simulink model "ScriptSimulinkVersion"  (R2023a)
settings: Solver=VariableStepAuto  StartTime=0.0  StopTime=t(end)  RelTol=1e-3
values from neighbouring files (symbols this model uses):
  Af = 2.2    [GPT_TrailerModelv3.m]
  Bx = 8    [GPT_TrailerModelv3.m]
  Bx_cap = 6    [GPT_TrailerModelv3.m]
  Cd = 0.8    [GPT_TrailerModelv3.m]
  Crr = 0.015    [GPT_TrailerModelv3.m]
  Cseat = diag([2e3, 8e3, 1.2e4])    [GPT_TrailerModelv3.m]
  ctc = 4.0e3    (= 4000)    [GPT_TrailerModelv3.m]
  Cx = 1.5    [GPT_TrailerModelv3.m]
  Cy = 7.5e4    (= 75000)    [GPT_TrailerModelv3.m]
  CyawM = 400    [GPT_TrailerModelv3.m]
  Dx = 0.8*2500    (= 2000)    [GPT_TrailerModelv3.m]
  epsv = 0.2    [GPT_TrailerModelv3.m]
  Ex = 0.0    (= 0)    [GPT_TrailerModelv3.m]
  g = 9.81    [GPT_TrailerModelv3.m]
  IAF = diag([20, 40, 40])    [GPT_TrailerModelv3.m]
  IB = diag([450, 2200, 2500])    [GPT_TrailerModelv3.m]
  Jw = 1.8    [GPT_TrailerModelv3.m]
  Kseat = diag([2e5, 5e5, 6e4])    [GPT_TrailerModelv3.m]
  ktc = 1.2e5    (= 120000)    [GPT_TrailerModelv3.m]
  mAF = 100    [GPT_TrailerModelv3.m]
  mAR = 110    [GPT_TrailerModelv3.m]
  mB = 1200    [GPT_TrailerModelv3.m]
  mu = 1.0    (= 1)    [GPT_TrailerModelv3.m]
  r_F_L_B = [axleF_x; +trackF/2; seat_zB]    [GPT_TrailerModelv3.m]
  r_F_R_B = [axleF_x; -trackF/2; seat_zB]    [GPT_TrailerModelv3.m]
  r_LF_A = [0; +trackF/2; 0]    [GPT_TrailerModelv3.m]
  r_LR_A = [0; +trackR/2; 0]    [GPT_TrailerModelv3.m]
  r_R_L_B = [axleR_x; +trackR/2; seat_zB]    [GPT_TrailerModelv3.m]
  r_R_R_B = [axleR_x; -trackR/2; seat_zB]    [GPT_TrailerModelv3.m]
  r_RF_A = [0; -trackF/2; 0]    [GPT_TrailerModelv3.m]
  r_RR_A = [0; -trackR/2; 0]    [GPT_TrailerModelv3.m]
  rho = 1.225    [GPT_TrailerModelv3.m]
  Rw = 0.35    [GPT_TrailerModelv3.m]
  tau_sync = 0.4    [GPT_TrailerModelv3.m]
  Tloss_c = 0.01    [GPT_TrailerModelv3.m]
  v_sync_on = 0.5    [GPT_TrailerModelv3.m]
  vblend = 0.5    [GPT_TrailerModelv3.m]
  Wind_E = [0;0;0]    [GPT_TrailerModelv3.m]
  x0 = [ rB0 ... (first row only)    [GPT_TrailerModelv3.m]
undefined symbols (not defined in the file or in its folder): P
settings Model: Creator=TEOMAN  LastModifiedBy=TEOMAN

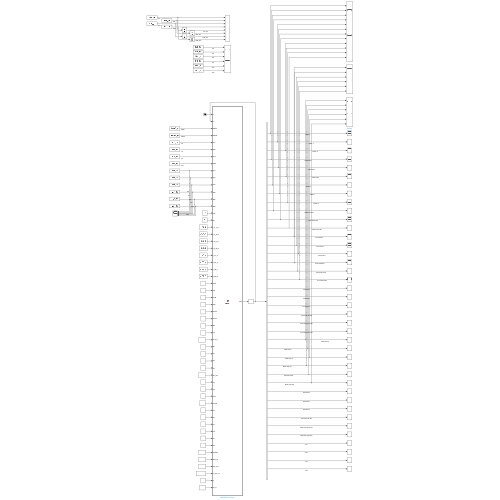
[thumbnail: Simulink's stored preview of the top-level diagram]
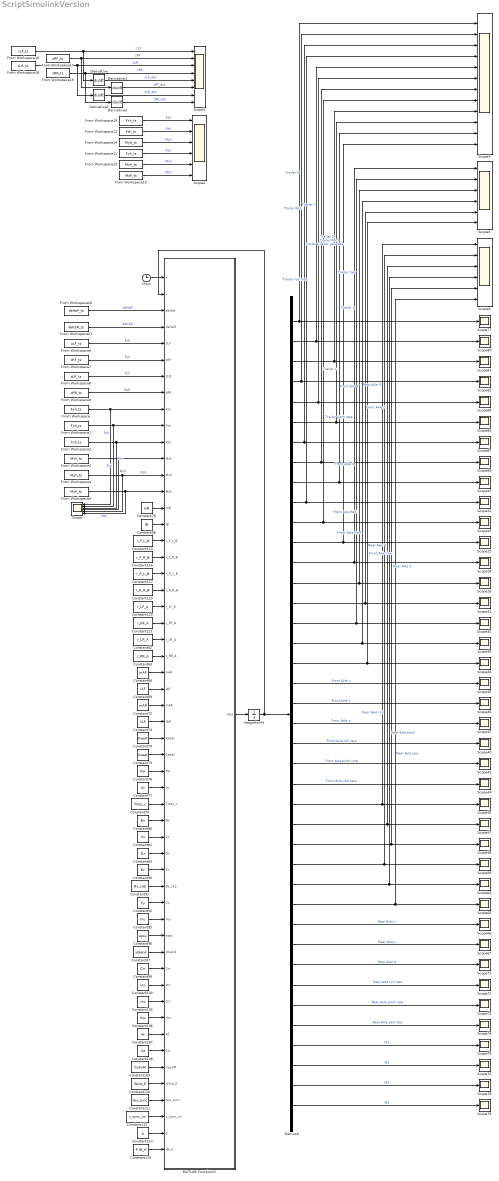
== system ScriptSimulinkVersion ==
  Clock : Clock
  Constant100 : Constant  Value=ktc
  Constant105 : Constant  Value=ctc
  Constant106 : Constant  Value=rho
  Constant107 : Constant  Value=Af
  Constant108 : Constant  Value=Cd
  Constant109 : Constant  Value=CyawM
  Constant110 : Constant  Value=Wind_E
  Constant111 : Constant  Value=tau_sync
  Constant112 : Constant  Value=v_sync_on
  Constant113 : Constant  Value=r_F_L_B
  Constant114 : Constant  Value=g
  Constant115 : Constant  Value=P.rB_H
  Constant116 : Constant  Value=r_F_R_B
  Constant117 : Constant  Value=r_R_L_B
  Constant119 : Constant  Value=r_R_R_B
  Constant120 : Constant  Value=r_LF_A
  Constant121 : Constant  Value=r_RF_A
  Constant62 : Constant  Value=r_LR_A
  Constant63 : Constant  Value=r_RR_A
  Constant66 : Constant  Value=mAF
  Constant69 : Constant  Value=IAF
  Constant72 : Constant  Value=mAR
  Constant73 : Constant  Value=IAF
  Constant74 : Constant  Value=Kseat
  Constant75 : Constant  Value=Cseat
  Constant76 : Constant  Value=Rw
  Constant77 : Constant  Value=Jw
  Constant78 : Constant  Value=mB
  Constant79 : Constant  Value=Tloss_c
  Constant80 : Constant  Value=Bx
  Constant81 : Constant  Value=Cx
  Constant83 : Constant  Value=Dx
  Constant90 : Constant  Value=Ex
  Constant91 : Constant  Value=Bx_cap
  Constant92 : Constant  Value=Cy
  Constant95 : Constant  Value=mu
  Constant96 : Constant  Value=epsv
  Constant97 : Constant  Value=vblend
  Constant98 : Constant  Value=IB
  Constant99 : Constant  Value=Crr
  Demux8 : Demux  Outputs=40
  Derivative{,1..3} (4 alike) : Derivative
  From Workspace : FromWorkspace  VariableName=Fxh_ts
  From Workspace1 : FromWorkspace  VariableName=Fyh_ts
  From Workspace10 : FromWorkspace  VariableName=Fxh_ts
  From Workspace11 : FromWorkspace  VariableName=Fyh_ts
  From Workspace12 : FromWorkspace  VariableName=Fzh_ts
  From Workspace13 : FromWorkspace  VariableName=Mxh_ts
  From Workspace14 : FromWorkspace  VariableName=Myh_ts
  From Workspace15 : FromWorkspace  VariableName=Mzh_ts
  From Workspace16 : FromWorkspace  VariableName=zLF_ts
  From Workspace17 : FromWorkspace  VariableName=zRF_ts
  From Workspace18 : FromWorkspace  VariableName=zLR_ts
  From Workspace19 : FromWorkspace  VariableName=zRR_ts
  From Workspace2 : FromWorkspace  VariableName=Fzh_ts
  From Workspace20 : FromWorkspace  VariableName=deltaF_ts
  From Workspace21 : FromWorkspace  VariableName=deltaR_ts
  From Workspace3 : FromWorkspace  VariableName=Mxh_ts
  From Workspace4 : FromWorkspace  VariableName=Myh_ts
  From Workspace5 : FromWorkspace  VariableName=Mzh_ts
  From Workspace6 : FromWorkspace  VariableName=zLF_ts
  From Workspace7 : FromWorkspace  VariableName=zRF_ts
  From Workspace8 : FromWorkspace  VariableName=zLR_ts
  From Workspace9 : FromWorkspace  VariableName=zRR_ts
  Integrator34 : Integrator  InitialCondition=x0
  MATLAB Function21 : MATLAB Function  TreatAsAtomicUnit=on
  Scope{,2,4..5} (4 alike) : Scope  NumInputPorts=6
  Scope1 : Scope  NumInputPorts=8
  Scope{20,22..23,25..26,28,31..37,40,43..44,56..59,64..67,71..82,84..85,87,89} (40 alike) : Scope
  Scope3 : Scope  NumInputPorts=12
  wires:
  From Workspace5/1 -> MATLAB Function21/14(Mzh), Scope/6  "Mzh"
  From Workspace/1 -> MATLAB Function21/9(Fxh), Scope/1  "Fxh"
  From Workspace3/1 -> MATLAB Function21/12(Mxh), Scope/4  "Mxh"
  Demux8/16 -> Scope5/2, Scope32/1  "Front Axle Roll"
  Demux8/23 -> Scope43/1  "Front Axle pitch rate"
  Integrator34/1 -> Demux8/1, MATLAB Function21/2(x)
  Demux8/13 -> Scope5/1, Scope26/1  "Front Axle X"
  Demux8/26 -> Scope4/3, Scope57/1  "Rear Axle Y"
  Demux8/6 -> Scope3/10, Scope85/1  "Trailer Yaw"
  Constant120/1 -> MATLAB Function21/21(r_LF_A)
  Constant69/1 -> MATLAB Function21/26(IAF)
  Constant75/1 -> MATLAB Function21/30(Cseat)
  Constant78/1 -> MATLAB Function21/15(mB)
  Demux8/35 -> Scope73/1  "Rear Axle pitch rate"
  Constant62/1 -> MATLAB Function21/23(r_LR_A)
  Constant63/1 -> MATLAB Function21/24(r_RR_A)
  Constant66/1 -> MATLAB Function21/25(mAF)
  Demux8/34 -> Scope72/1  "Rear Axle roll rate"
  Demux8/21 -> Scope37/1  "Front Axle w"
  Constant117/1 -> MATLAB Function21/19(r_R_L_B)
  Demux8/39 -> Scope78/1  "W3"
  Constant90/1 -> MATLAB Function21/37(Ex)
  MATLAB Function21/1(xdot) -> Integrator34/1
  Demux8/4 -> Scope3/2, Scope82/1  "Trailer Roll"
  Constant113/1 -> MATLAB Function21/17(r_F_L_B)
  Demux8/5 -> Scope3/6, Scope84/1  "Trailer Pitch"
  Constant72/1 -> MATLAB Function21/27(mAR)
  Constant116/1 -> MATLAB Function21/18(r_F_R_B)
  Demux8/15 -> Scope5/5, Scope31/1  "Front Axle Z"
  Demux8/27 -> Scope4/5, Scope58/1  "Rear Axle Z"
  Constant98/1 -> MATLAB Function21/16(IB)
  Constant74/1 -> MATLAB Function21/29(Kseat)
  Demux8/18 -> Scope34/1, Scope5/6  "Front Axle Yaw"
  Constant105/1 -> MATLAB Function21/45(ctc)
  Demux8/40 -> Scope79/1  "W4"
  Constant119/1 -> MATLAB Function21/20(r_R_R_B)
  Constant106/1 -> MATLAB Function21/46(rho)
  Demux8/33 -> Scope71/1  "Rear Axle w"
  Constant107/1 -> MATLAB Function21/47(Af)
  Demux8/29 -> Scope4/4, Scope64/1  "Rear Axle pitch"
  Demux8/30 -> Scope4/6, Scope65/1  "Rear Axle yaw"
  Constant121/1 -> MATLAB Function21/22(r_RF_A)
  Constant91/1 -> MATLAB Function21/38(Bx_cap)
  Demux8/24 -> Scope44/1  "Front Axle yaw rate"
  From Workspace4/1 -> MATLAB Function21/13(Myh), Scope/5  "Myh"
  Constant79/1 -> MATLAB Function21/33(Tloss_c)
  Constant114/1 -> MATLAB Function21/53(g)
  Constant80/1 -> MATLAB Function21/34(Bx)
  Demux8/38 -> Scope76/1  "W2"
  Constant96/1 -> MATLAB Function21/41(epsv)
  Demux8/7 -> Scope3/3, Scope87/1  "Trailer u"
  Demux8/2 -> Scope3/5, Scope80/1  "Trailer Y"
  Demux8/25 -> Scope4/1, Scope56/1  "Rear Axle X"
  Demux8/14 -> Scope28/1, Scope5/3  "Front Axle Y"
  Demux8/8 -> Scope3/7, Scope89/1  "Trailer v"
  Constant77/1 -> MATLAB Function21/32(Jw)
  Demux8/22 -> Scope40/1  "Front Axle roll rate"
  Demux8/9 -> Scope3/11, Scope20/1  "Trailer w"
  Constant92/1 -> MATLAB Function21/39(Cy)
  Demux8/11 -> Scope3/8, Scope23/1  "Trailer pitch rate"
  Demux8/28 -> Scope4/2, Scope59/1  "Rear Axle roll"
  Demux8/36 -> Scope74/1  "Rear Axle yaw rate"
  Demux8/37 -> Scope75/1  "W1"
  Demux8/32 -> Scope67/1  "Rear Axle v"
  Constant100/1 -> MATLAB Function21/44(ktc)
  Demux8/10 -> Scope3/4, Scope22/1  "Trailer roll rate"
  From Workspace1/1 -> MATLAB Function21/10(Fyh), Scope/2  "Fyh"
  Constant111/1 -> MATLAB Function21/51(tau_sync)
  Constant73/1 -> MATLAB Function21/28(IAR)
  Constant99/1 -> MATLAB Function21/43(Crr)
  Constant95/1 -> MATLAB Function21/40(mu)
  Constant115/1 -> MATLAB Function21/54(rB_H)
  Demux8/31 -> Scope66/1  "Rear Axle u"
  Constant76/1 -> MATLAB Function21/31(Rw)
  Demux8/3 -> Scope81/1, Scope3/9  "Trailer Z"
  Demux8/12 -> Scope3/12, Scope25/1  "Trailer yaw rate"
  From Workspace2/1 -> MATLAB Function21/11(Fzh), Scope/3  "Fzh"
  Demux8/17 -> Scope5/4, Scope33/1  "Front Axle Pitch"
  Clock/1 -> MATLAB Function21/1(t)
  Constant83/1 -> MATLAB Function21/36(Dx)
  Constant81/1 -> MATLAB Function21/35(Cx)
  Demux8/20 -> Scope36/1  "Front Axle v"
  Demux8/19 -> Scope35/1  "Front Axle u"
  Demux8/1 -> Scope3/1, Scope77/1  "Trailer X"
  Constant108/1 -> MATLAB Function21/48(Cd)
  Constant109/1 -> MATLAB Function21/49(CyawM)
  Constant110/1 -> MATLAB Function21/50(Wind_E)
  Constant97/1 -> MATLAB Function21/42(vblend)
  Constant112/1 -> MATLAB Function21/52(v_sync_on)
  From Workspace9/1 -> MATLAB Function21/8(zRR)  "Mxh"
  From Workspace8/1 -> MATLAB Function21/7(zLR)  "Fzh"
  From Workspace7/1 -> MATLAB Function21/6(zRF)  "Fyh"
  From Workspace6/1 -> MATLAB Function21/5(zLF)  "Fxh"
  From Workspace10/1 -> Scope2/1  "Fxh"
  From Workspace16/1 -> Derivative/1, Scope1/1  "zLF"
  Derivative/1 -> Scope1/5  "zLF_dot"
  From Workspace17/1 -> Derivative1/1, Scope1/2  "zRF"
  From Workspace19/1 -> Derivative3/1, Scope1/4  "zRR"
  From Workspace18/1 -> Derivative2/1, Scope1/3  "zLR"
  Derivative1/1 -> Scope1/6  "zRF_dot"
  Derivative2/1 -> Scope1/7  "zLR_dot"
  Derivative3/1 -> Scope1/8  "zRR_dot"
  From Workspace12/1 -> Scope2/2  "Fzh"
  From Workspace14/1 -> Scope2/3  "Myh"
  From Workspace11/1 -> Scope2/4  "Fyh"
  From Workspace13/1 -> Scope2/5  "Mxh"
  From Workspace15/1 -> Scope2/6  "Mzh"
  From Workspace20/1 -> MATLAB Function21/3(deltaF)  "deltaF"
  From Workspace21/1 -> MATLAB Function21/4(deltaR)  "deltaR"

== matlab function ScriptSimulinkVersion/MATLAB Function21 ==
  data: t input; xdot output; x input; deltaF input; deltaR input; zLF input; zRF input; zLR input; zRR input; Fxh input; Fyh input; Fzh input; Mxh input; Myh input; Mzh input; mB input; IB input; r_F_L_B input; r_F_R_B input; r_R_L_B input; r_R_R_B input; r_LF_A input; r_RF_A input; r_LR_A input; r_RR_A input; mAF input; IAF input; mAR input; IAR input; Kseat input; Cseat input; Rw input; Jw input; Tloss_c input; Bx input; Cx input; Dx input; Ex input; Bx_cap input; Cy input; mu input; epsv input; vblend input; Crr input; ktc input; ctc input; rho input; Af input; Cd input; CyawM input; Wind_E input; tau_sync input; v_sync_on input; g input; rB_H input
function xdot = TrailerBlock(t, x, ...
    deltaF, deltaR, zLF, zRF, zLR, zRR, ...
    Fxh, Fyh, Fzh, Mxh, Myh, Mzh, ...
    mB, IB, ...
    r_F_L_B, r_F_R_B, r_R_L_B, r_R_R_B, ...
    r_LF_A, r_RF_A, r_LR_A, r_RR_A, ...
    mAF, IAF, mAR, IAR, Kseat, Cseat, ...
    Rw, Jw, Tloss_c, ...
    Bx, Cx, Dx, Ex, Bx_cap, Cy, mu, epsv, vblend, Crr, ...
    ktc, ctc, ...
    rho, Af, Cd, CyawM, Wind_E, ...
    tau_sync, v_sync_on, g, rB_H)

% ================== UNPACK STATES ========================================
i = 1;
% Body
rB = x(i:i+2);  i = i+3;
phiB   = x(i); thetaB = x(i+1); psiB = x(i+2); i = i+3;
vB = x(i:i+2); i = i+3;
wB = x(i:i+2); i = i+3;

% Front axle
rAF = x(i:i+2); i = i+3;
phiAF   = x(i); thetaAF = x(i+1); psiAF = x(i+2); i = i+3;
vAF = x(i:i+2); i = i+3;
wAF = x(i:i+2); i = i+3;

% Rear axle
rAR = x(i:i+2); i = i+3;
phiAR   = x(i); thetaAR = x(i+1); psiAR = x(i+2); i = i+3;
vAR = x(i:i+2); i = i+3;
wAR = x(i:i+2); i = i+3;

% Wheel spins
omegaLF = x(i); omegaRF = x(i+1); omegaLR = x(i+2); omegaRR = x(i+3);

% ================== ROTATION MATRICES ====================================
RB  = eulZYX_to_R(phiB,thetaB,psiB); %RB = eye(3);
RAF = eulZYX_to_R(phiAF,thetaAF,psiAF); %RAF = eye(3);
RAR = eulZYX_to_R(phiAR,thetaAR,psiAR); %RAR = eye(3);

% ================== BUSHINGS (BODY–AXLE) =================================
[Fb_B, Mb_B, F_F_A, M_F_A, F_R_A, M_R_A] = ...
    two_point_bushings(rB,vB,wB,RB, ...
                       rAF,vAF,wAF,RAF, ...
                       rAR,vAR,wAR,RAR, ...
                       r_F_L_B,r_F_R_B,r_R_L_B,r_R_R_B, ...
                       r_LF_A,r_RF_A,r_LR_A,r_RR_A, ...
                       Kseat,Cseat);

% ================== WHEEL KINEMATICS =====================================
[pLF_E,vLF_E] = wheel_kin(rAF,RAF,vAF,wAF,r_LF_A);
[pRF_E,vRF_E] = wheel_kin(rAF,RAF,vAF,wAF,r_RF_A);
[pLR_E,vLR_E] = wheel_kin(rAR,RAR,vAR,wAR,r_LR_A);
[pRR_E,vRR_E] = wheel_kin(rAR,RAR,vAR,wAR,r_RR_A);

% ================== VERTICAL TIRE FORCES =================================
FzLF = tire_normal_soft(pLF_E(3), vLF_E(3), zLF, Rw, ktc, ctc);
FzRF = tire_normal_soft(pRF_E(3), vRF_E(3), zRF, Rw, ktc, ctc);
FzLR = tire_normal_soft(pLR_E(3), vLR_E(3), zLR, Rw, ktc, ctc);
FzRR = tire_normal_soft(pRR_E(3), vRR_E(3), zRR, Rw, ktc, ctc);

% ================== TIRE FORCES (MAGIC FORMULA) ==========================
[FxLF_A,FyLF_A,FxLF_w,vxLF_w] = tire_forces_MF(vLF_E,RAF,deltaF,omegaLF,FzLF, ...
    Rw,Bx,Cx,Dx,Ex,Bx_cap,Cy,mu,epsv,vblend,Crr);
[FxRF_A,FyRF_A,FxRF_w,vxRF_w] = tire_forces_MF(vRF_E,RAF,deltaF,omegaRF,FzRF, ...
    Rw,Bx,Cx,Dx,Ex,Bx_cap,Cy,mu,epsv,vblend,Crr);
[FxLR_A,FyLR_A,FxLR_w,vxLR_w] = tire_forces_MF(vLR_E,RAR,deltaR,omegaLR,FzLR, ...
    Rw,Bx,Cx,Dx,Ex,Bx_cap,Cy,mu,epsv,vblend,Crr);
[FxRR_A,FyRR_A,FxRR_w,vxRR_w] = tire_forces_MF(vRR_E,RAR,deltaR,omegaRR,FzRR, ...
    Rw,Bx,Cx,Dx,Ex,Bx_cap,Cy,mu,epsv,vblend,Crr);

% Friction ellipse (same as original ode_trailer)
[FxLF_A,FyLF_A] = friction_ellipse_smooth(FxLF_A,FyLF_A,FzLF,mu);
[FxRF_A,FyRF_A] = friction_ellipse_smooth(FxRF_A,FyRF_A,FzRF,mu);
[FxLR_A,FyLR_A] = friction_ellipse_smooth(FxLR_A,FyLR_A,FzLR,mu);
[FxRR_A,FyRR_A] = friction_ellipse_smooth(FxRR_A,FyRR_A,FzRR,mu);

% ================== WHEEL-FRAME LONGITUDINAL (FOR TORQUE) ================
cF = cos(deltaF); sF = sin(deltaF);
cR = cos(deltaR); sR = sin(deltaR);

FxLF_w_t =  cF*FxLF_A + sF*FyLF_A;
FxRF_w_t =  cF*FxRF_A + sF*FyRF_A;
FxLR_w_t =  cR*FxLR_A + sR*FyLR_A;
FxRR_w_t =  cR*FxRR_A + sR*FyRR_A;

% ================== AXLE RESULTANTS ======================================
FzLF_A = RAF'*[0;0;FzLF];
FzRF_A = RAF'*[0;0;FzRF];
FzLR_A = RAR'*[0;0;FzLR];
FzRR_A = RAR'*[0;0;FzRR];

FwLF_A = [FxLF_A;FyLF_A;0] + FzLF_A;
FwRF_A = [FxRF_A;FyRF_A;0] + FzRF_A;
FwLR_A = [FxLR_A;FyLR_A;0] + FzLR_A;
FwRR_A = [FxRR_A;FyRR_A;0] + FzRR_A;

F_axF_A = F_F_A + FwLF_A + FwRF_A;
M_axF_A = M_F_A + cross3(r_LF_A,FwLF_A) + cross3(r_RF_A,FwRF_A);
F_axR_A = F_R_A + FwLR_A + FwRR_A;
M_axR_A = M_R_A + cross3(r_LR_A,FwLR_A) + cross3(r_RR_A,FwRR_A);

% ================== BODY FORCES / MOMENTS ================================
Fg_B    = RB'*[0;0;-mB*g];                        % gravity in body frame
% Fg_B =  [0;0;-mB*g];
Faero_B = aero_body(vB,RB,Wind_E,rho,Af,Cd);      % aero in body frame
Maero_B = [0;0;-CyawM*vB(2)];                     % yaw aero moment

F_body_B = Fb_B + Fg_B + Faero_B;
M_body_B = Mb_B + Maero_B;

% Hitch loads (already in body frame here)
Fh_B = [Fxh; Fyh; Fzh];
Mh_B = [Mxh; Myh; Mzh];

M_hitch_total = Mh_B + cross3(rB_H, Fh_B);

F_body_B = F_body_B + Fh_B;
M_body_B = M_body_B + M_hitch_total;

% ================== BODY DYNAMICS ========================================
vBd  = (F_body_B - cross3(wB,mB*vB))/mB;
wBd  = IB \ ( M_body_B - cross3(wB,IB*wB) );
rBd  = RB * vB;
eBdot = eulRatesZYX_from_bodyRates(phiB,thetaB,wB);

% ================== FRONT AXLE DYNAMICS ==================================
Fg_AF_A = RAF'*[0;0;-mAF*g]; %Fg_AF_A =[0;0;-mAF*g];
vAFd = (F_axF_A + Fg_AF_A - cross3(wAF,mAF*vAF))/mAF;
wAFd = IAF \ (M_axF_A - cross3(wAF,IAF*wAF));
rAFd = RAF*vAF;
eAFdot = eulRatesZYX_from_bodyRates(phiAF,thetaAF,wAF);

% ================== REAR AXLE DYNAMICS ===================================
Fg_AR_A = RAR'*[0;0;-mAR*g]; %Fg_AR_A = [0;0;-mAR*g];
vARd = (F_axR_A + Fg_AR_A - cross3(wAR,mAR*vAR))/mAR;
wARd = IAR \ (M_axR_A - cross3(wAR,IAR*wAR));
rARd = RAR*vAR;
eARdot = eulRatesZYX_from_bodyRates(phiAR,thetaAR,wAR);

% ================== WHEEL-SPIN ODEs (NO BRAKES HERE) =====================
TbLF = 0; TbRF = 0; TbLR = 0; TbRR = 0;   % or pass as inputs later

omegaLFd = ( FxLF_w_t*Rw - TbLF - Tloss_c*omegaLF ) / Jw;
omegaRFd = ( FxRF_w_t*Rw - TbRF - Tloss_c*omegaRF ) / Jw;
omegaLRd = ( FxLR_w_t*Rw - TbLR - Tloss_c*omegaLR ) / Jw;
omegaRRd = ( FxRR_w_t*Rw - TbRR - Tloss_c*omegaRR ) / Jw;

% ================== SYNC CORRECTION (MATCHES ode_trailer) ================
gainL  = 0.5*(v_sync_on / sqrt(vxLF_w*vxLF_w + v_sync_on^2));
gainR  = 0.5*(v_sync_on / sqrt(vxRF_w*vxRF_w + v_sync_on^2));
gainLR = 0.5*(v_sync_on / sqrt(vxLR_w*vxLR_w + v_sync_on^2));
gainRR = 0.5*(v_sync_on / sqrt(vxRR_w*vxRR_w + v_sync_on^2));

omegaLFd = omegaLFd + gainL *((vxLF_w/Rw) - omegaLF)/tau_sync;
omegaRFd = omegaRFd + gainR *((vxRF_w/Rw) - omegaRF)/tau_sync;
omegaLRd = omegaLRd + gainLR*((vxLR_w/Rw) - omegaLR)/tau_sync;
omegaRRd = omegaRRd + gainRR*((vxRR_w/Rw) - omegaRR)/tau_sync;

% ================== OUTPUT STATE DERIVATIVE ==============================
xdot = [ rBd; eBdot; vBd; wBd; ...
         rAFd; eAFdot; vAFd; wAFd; ...
         rARd; eARdot; vARd; wARd; ...
         omegaLFd; omegaRFd; omegaLRd; omegaRRd ];
end

%% =================== SUPPORT FUNCTIONS ==================================
function [Fb_B, Mb_B, F_F_A, M_F_A, F_R_A, M_R_A] = ...
    two_point_bushings(rB,vB,wB,RB, ...
                       rAF,vAF,wAF,RAF, ...
                       rAR,vAR,wAR,RAR, ...
                       r_F_L_B,r_F_R_B,r_R_L_B,r_R_R_B, ...
                       r_LF_A,r_RF_A,r_LR_A,r_RR_A, ...
                       Kseat,Cseat)

Fb_B = [0;0;0]; Mb_B = [0;0;0];
F_F_A = [0;0;0]; M_F_A = [0;0;0];
F_R_A = [0;0;0]; M_R_A = [0;0;0];

[fb1,mb1,f1,m1] = seat(rB,r_F_L_B,RB,vB,wB, rAF,r_LF_A,RAF,vAF,wAF,Kseat,Cseat);
[fb2,mb2,f2,m2] = seat(rB,r_F_R_B,RB,vB,wB, rAF,r_RF_A,RAF,vAF,wAF,Kseat,Cseat);

Fb_B = Fb_B+fb1+fb2;  Mb_B = Mb_B+mb1+mb2;
F_F_A=F_F_A+f1+f2;    M_F_A=M_F_A+m1+m2;

[fb3,mb3,f3,m3] = seat(rB,r_R_L_B,RB,vB,wB, rAR,r_LR_A,RAR,vAR,wAR,Kseat,Cseat);
[fb4,mb4,f4,m4] = seat(rB,r_R_R_B,RB,vB,wB, rAR,r_RR_A,RAR,vAR,wAR,Kseat,Cseat);

Fb_B = Fb_B+fb3+fb4; Mb_B = Mb_B+mb3+mb4;
F_R_A=F_R_A+f3+f4;   M_R_A=M_R_A+m3+m4;
end

function [Fb_B,Mb_B,F_A,M_A] = seat(rB,rSeatB,RB,vB,wB, ...
                                    rA,rSeatA,RA,vA,wA, K,C)
pB = rB + RB*rSeatB;
vB_ = RB*(vB + cross3(wB,rSeatB));
pA = rA + RA*rSeatA;
vA_ = RA*(vA + cross3(wA,rSeatA));

d  = RB'*(pA - pB);
vd = RB'*(vA_ - vB_);

F_B = K*d + C*vd;
M_B = cross3(rSeatB,F_B);

Fb_B = F_B;
Mb_B = M_B;
F_A  = RA'*(-RB*F_B);
M_A  = cross3(rSeatA,F_A);
end

function [p,v] = wheel_kin(rA,RA,vA,wA,r)
p = rA + RA*r;
v = RA*(vA + cross3(wA,r));
end

function Fz = tire_normal_soft(zW,zWdot,zRoad,Rw,ktc,ctc)
comp = (zRoad + Rw) - zW;
hc   = 0.5*(comp + sqrt(comp*comp + 1e-6));      % smooth ReLU
gate = 0.5*(1 + comp/sqrt(comp*comp + 1e-6));    % ~1 in contact
Fz   = ktc*hc + ctc*gate*max(0,-zWdot);          % no pull on rebound
end

function [Fx_A,Fy_A,Fx_w,vx_w] = tire_forces_MF(vWheel_E,RA,delta,omega,Fz, ...
    Rw,Bx,Cx,Dx,Ex,Bx_cap,Cy,mu,epsv,vblend,Crr)

% to axle frame
vA = RA'*vWheel_E;

c = cos(delta); s = sin(delta);
vx_w =  c*vA(1) + s*vA(2);
vy_w = -s*vA(1) + c*vA(2);

vx_abs = sqrt(vx_w*vx_w + epsv^2);
b      = vx_abs/(vx_abs + vblend);

lam = (vx_w - Rw*omega) / vx_abs;     % same sign as original ode_trailer
% lam = (Rw*omega - vx_w) / vx_abs;
lam = min(max(lam,-1),1);
lam = b*lam;

alpha = b*atan2(vy_w, vx_abs);

Bx_eff = min(Bx,Bx_cap);
phi    = Bx_eff*lam;
Fx_star = Dx * sin( Cx * atan( phi - Ex*(phi - atan(phi)) ) );

Fy_star = -Cy*alpha;

sig     = vx_w / sqrt(vx_w*vx_w + (0.2*vblend)^2);
Fx_star = Fx_star - Crr*Fz*sig;

Fx_A =  c*Fx_star - s*Fy_star;
Fy_A =  s*Fx_star + c*Fy_star;

Fx_w = Fx_star;
end

function [Fx,Fy] = friction_ellipse_smooth(Fx,Fy,Fz,mu)
Flim = max(mu*Fz,1e-3);
mag  = hypot(Fx,Fy) + 1e-12;
if mag>Flim
    s = Flim/mag;
    Fx = Fx*s; Fy = Fy*s;
end
end

function Faero_B = aero_body(vB_B, RB_E, Wind_E, rho, Af, Cd)
Vrel_B = vB_B - (RB_E'*Wind_E);
Va = norm(Vrel_B);
if Va > 0
    Faero_B = -0.5*rho*Af*Cd*Va*Vrel_B;
else
    Faero_B = [0;0;0];
end
end

function C = cross3(a,b)
C=[a(2)*b(3)-a(3)*b(2);
   a(3)*b(1)-a(1)*b(3);
   a(1)*b(2)-a(2)*b(1)];
end

function R = eulZYX_to_R(phi,theta,psi)
c1=cos(phi); s1=sin(phi);
c2=cos(theta); s2=sin(theta);
c3=cos(psi); s3=sin(psi);
R=[ c3*c2,             c3*s2*s1 - s3*c1,   c3*s2*c1 + s3*s1;
    s3*c2,             s3*s2*s1 + c3*c1,   s3*s2*c1 - c3*s1;
    -s2,               c2*s1,              c2*c1 ];
end

function e = eulRatesZYX_from_bodyRates(phi,theta,w)
p=w(1); q=w(2); r=w(3);
c1=cos(phi); s1=sin(phi);
c2=cos(theta); s2=sin(theta);
if abs(c2)<1e-6, c2=sign(c2)*1e-6; end
t2=s2/c2;
e=[1, s1*t2, c1*t2;
   0, c1,   -s1;
   0, s1/c2, c1/c2]*[p;q;r];
end
